simulink model "modelo_p1_2023"  (R2025a)
settings: Solver=VariableStepAuto  StartTime=0.0  StopTime=10.0  RelTol=1e-3
settings Model: Creator=joaof  LastModifiedBy=joaof

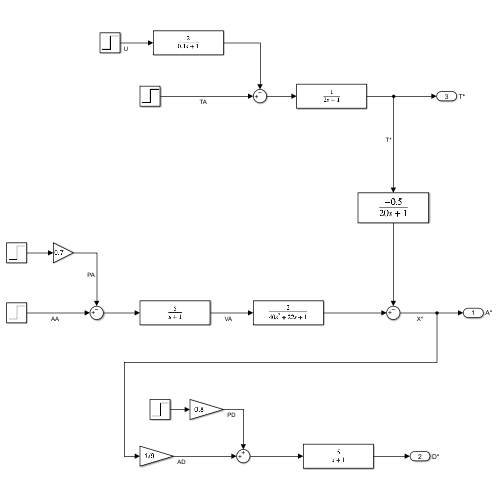
[thumbnail: Simulink's stored preview of the top-level diagram]
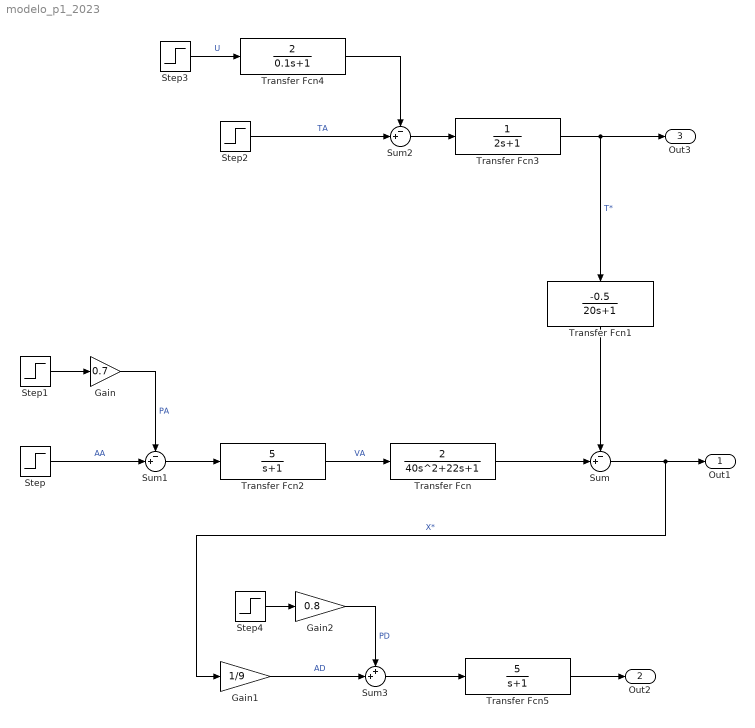
== system modelo_p1_2023 ==
  Gain : Gain  Gain=0.7
  Gain1 : Gain  Gain=1/9
  Gain2 : Gain  Gain=0.8
  Step{,1..4} (5 alike) : Step  SampleTime=0
  Sum : Sum  Inputs=-+|
  Sum1 : Sum  Inputs=-+|
  Sum2 : Sum  Inputs=-+|
  Sum3 : Sum  Inputs=++|
  Transfer Fcn : TransferFcn  Numerator=[2]  Denominator=[40 22 1]
  Transfer Fcn1 : TransferFcn  Numerator=[-0.5]  Denominator=[20 1]
  Transfer Fcn2 : TransferFcn  Numerator=[5]  Denominator=[1 1]
  Transfer Fcn3 : TransferFcn  Denominator=[2 1]
  Transfer Fcn4 : TransferFcn  Numerator=[2]  Denominator=[0.1 1]
  Transfer Fcn5 : TransferFcn  Numerator=[5]  Denominator=[1 1]
  Out1 : Outport  SignalName=A*
  Out2 : Outport  Port=2  SignalName=D*
  Out3 : Outport  Port=3  SignalName=T*
  wires:
  Transfer Fcn1/1 -> Sum/1
  Sum/1 -> Gain1/1, Out1/1  "X*"
  Transfer Fcn/1 -> Sum/2
  Transfer Fcn2/1 -> Transfer Fcn/1  "VA"
  Step1/1 -> Gain/1
  Sum1/1 -> Transfer Fcn2/1
  Step/1 -> Sum1/2  "AA"
  Gain/1 -> Sum1/1  "PA"
  Transfer Fcn3/1 -> Out3/1, Transfer Fcn1/1  "T*"
  Sum2/1 -> Transfer Fcn3/1
  Transfer Fcn4/1 -> Sum2/1
  Step2/1 -> Sum2/2  "TA"
  Step3/1 -> Transfer Fcn4/1  "U"
  Gain1/1 -> Sum3/2  "AD"
  Step4/1 -> Gain2/1
  Gain2/1 -> Sum3/1  "PD"
  Sum3/1 -> Transfer Fcn5/1
  Transfer Fcn5/1 -> Out2/1
